simulink model "controller"  (R2016a)
settings: Solver=VariableStepAuto  StartTime=0.0  StopTime=10.0  RelTol=1e-3
values from neighbouring files (symbols this model uses):
  Xkk = Cin(N*p+N+1:end)    [Controller.m]
  Ymeas = Cin(N*p+1:N*p+N)    [Controller.m]    (also in sample.mat = [2 2 200])
  Yref = reshape(Cin(1:N*p),N,[])    [Controller.m]
settings Model: Creator=hp  LastModifiedBy=hp

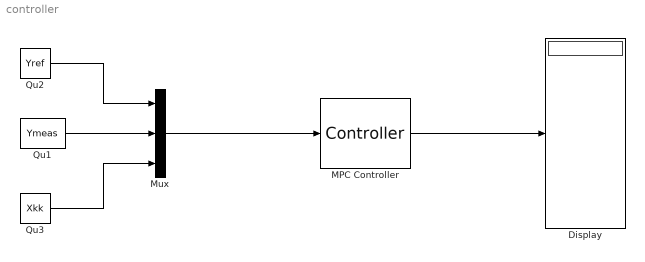
== system controller ==
  Display : Display
  MPC Controller : MATLABFcn  MATLABFcn=Controller  Output1D=off
  Mux : Mux  Inputs=3
  Qu1 : Constant  Value=Ymeas  VectorParams1D=off
  Qu2 : Constant  Value=Yref  VectorParams1D=off
  Qu3 : Constant  Value=Xkk  VectorParams1D=off
  wires:
  Qu2/1 -> Mux/1
  Qu1/1 -> Mux/2
  Qu3/1 -> Mux/3
  Mux/1 -> MPC Controller/1
  MPC Controller/1 -> Display/1
